simulink model "Simple_CameraInputDisplay_UCS"  (R2025b)
settings: Solver=FixedStepDiscrete  StartTime=0.0  StopTime=inf  FixedStep=.01  RelTol=1e-3
model workspace (MAT data in the model file):
  socvcb = containers.Map
  socvcb.serialization.keys = {}
  socvcb.serialization.values = {}
  socvcb.serialization.uniformity = 0
  socvcb.serialization.keyType = 'double'
  socvcb.serialization.valueType = 'any'
undefined symbols (not defined in the file): distort_coefL, gate1_Pose, gray, k_L, keyPointsWorld, M_UCSToWorld, M_WorldToUCS, numKeypoints, rel_CamPose_L, rel_CamPose_L_UCS, rel_CamPose_R_UCS, Sim3dSensor
libraries: sim3dlib x3, sim3dcameralib x2, visionsinks x2, visiontextngfix x1, visionconversions x1
settings Model: Creator=Liam  LastModifiedBy=Liam

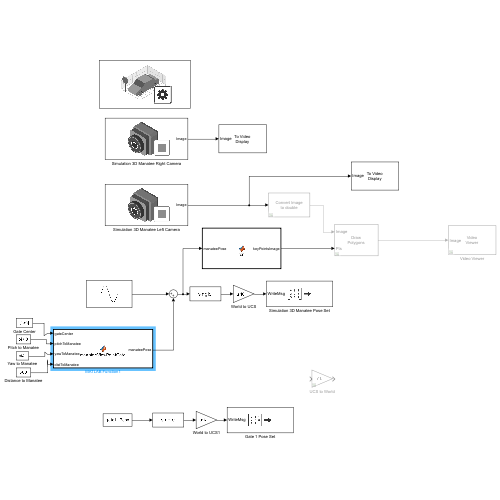
[thumbnail: Simulink's stored preview of the top-level diagram]
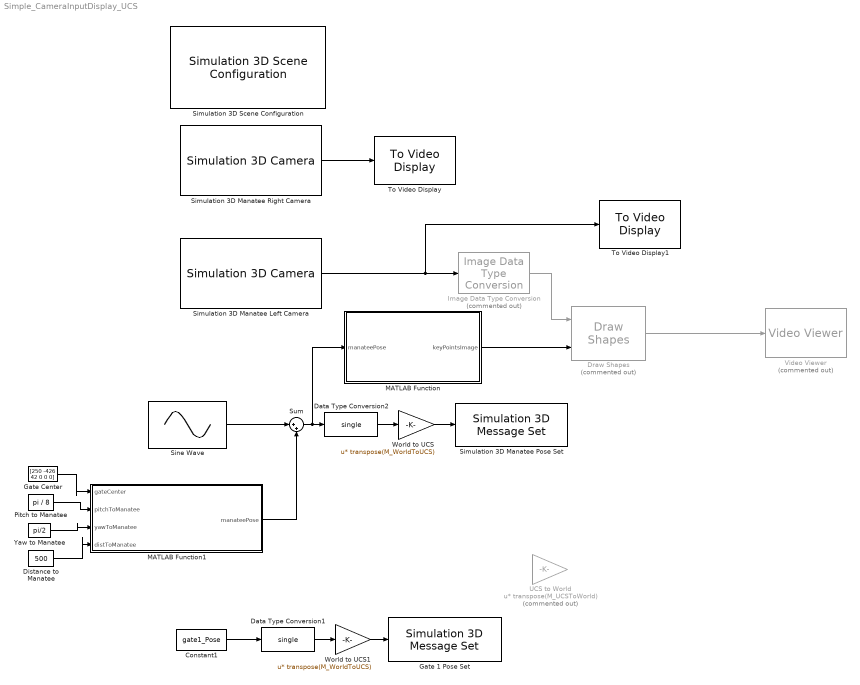
== system Simple_CameraInputDisplay_UCS ==
  Constant1 : Constant  Value=gate1_Pose  VectorParams1D=off  OutDataTypeStr=single
  Data Type Conversion1 : DataTypeConversion  OutDataTypeStr=single  SaturateOnIntegerOverflow=off  RndMeth=Floor
  Data Type Conversion2 : DataTypeConversion  OutDataTypeStr=single  SaturateOnIntegerOverflow=off  RndMeth=Floor
  Distance to Manatee : Constant  Value=500
  Draw Shapes : visiontextngfix/Draw Shapes  Commented=on  shape=Polygons  fill=off  lineWidth=2  fillClrSource=Specify via dialog  display=User-specified value  intensity=200  color=[255 255 0]  opacity=0.6  viewport=Entire image  antialiasing=off  inType=Obsolete  imagePorts=One multidimensional signal  roundingMode=Floor  overflowMode=off  memoryMode=Specify word length  memoryWordLength=16  prodOutputMode=Binary point scaling  prodOutputWordLength=32  prodOutputFracLength=14  memoryFracLength=15
  Gate 1 Pose Set : sim3dlib/Simulation 3D Message Set  Priority=-1  SigName=Gate1PoseSet  Ts=-1  aMode=0
      settings: LibrarySourceBlock=aerolibsim3d/Simulation 3D Message Set
  Gate Center : Constant  Value=[250 -426 42 0 0 0]  VectorParams1D=off  OutDataTypeStr=single
  Image Data Type Conversion : visionconversions/Image Data Type Conversion  Commented=on  outDT=double  isSigned=on  wordLen=16  numFracBits=0
  MATLAB Function : MATLAB Function  TreatAsAtomicUnit=on
  MATLAB Function1 : MATLAB Function  TreatAsAtomicUnit=on
  Pitch to Manatee : Constant  Value=pi / 8
  Simulation 3D Manatee Left Camera : sim3dcameralib/Simulation 3D Camera  Priority=1  sensorTag=Sim3dSensor�  sensorId=1  sensorName=Sim3dSensor�  vehTagList={'Scene Origin'}  vehTag=Scene Origin  CoordinateSystem=Default  mountLoc=Origin  offsetFlag=on  tmountOffset=rel_CamPose_L_UCS(1:3) / 100  extTmount=off  rmountOffset=rel_CamPose_L_UCS(4:6)  extRmount=off  FocalLength=[2.97 / 0.0028, 2.97 / 0.0028]  OpticalCenter=[960, 540]  ImageSize=[1080, 1920]  RadialDistortion=[0.30 0.08]  TangentialDistortion=[0 0]  SensorSkew=0  VisualizeFieldOfView=off  FieldOfViewRange=61  DepthOutportEnabled=off  SemanticOutportEnabled=off  TransformOutportEnabled=off  SampleTime=-1  mountPoint=[0.4 -0.125 -0.15]  mountOrientation=[0 0 0]  aMode=5  ID=1
      settings: LibrarySourceBlock=sl3dlib/Simulation 3D/Sensors/Simulation 3D Camera
  Simulation 3D Manatee Pose Set : sim3dlib/Simulation 3D Message Set  Priority=-1  SigName=ManateePoseSet  Ts=-1  aMode=0
      settings: LibrarySourceBlock=aerolibsim3d/Simulation 3D Message Set
  Simulation 3D Manatee Right Camera : sim3dcameralib/Simulation 3D Camera  Priority=1  sensorTag=Sim3dSensor�  sensorId=2  sensorName=Sim3dSensor�  vehTagList={'Scene Origin'}  vehTag=Scene Origin  CoordinateSystem=Default  mountLoc=Origin  offsetFlag=on  tmountOffset=rel_CamPose_R_UCS(1:3) / 100  extTmount=off  rmountOffset=rel_CamPose_R_UCS(4:6)  extRmount=off  FocalLength=[2.97 / 0.0028, 2.97 / 0.0028]  OpticalCenter=[960, 540]  ImageSize=[1080, 1920]  RadialDistortion=[0.30 0.08]  TangentialDistortion=[0 0]  SensorSkew=0  VisualizeFieldOfView=off  FieldOfViewRange=61  DepthOutportEnabled=off  SemanticOutportEnabled=off  TransformOutportEnabled=off  SampleTime=-1  mountPoint=[0.4 0.125 -0.15]  mountOrientation=[0 0 0]  aMode=5  ID=2
      settings: LibrarySourceBlock=sl3dlib/Simulation 3D/Sensors/Simulation 3D Camera
  Simulation 3D Scene Configuration : sim3dlib/Simulation 3D Scene Configuration  Priority=0  ProjectFormat=Unreal Executable  SceneDesc=Straight road  ProjectName=C:\Users\Liam\OneDrive\Documents\GitHub\Vision_Sim\Unreal\UnrealProjects\SimulinkCoSimulation\EllingtonPoolSim\Windows\EllingtonPoolSim.exe  ScenePath=/Game/PoolMapQuickWater  UEProjPath=C:\Users\Liam\OneDrive\Documents\GitHub\Vision_Sim\Unreal\UnrealProjects\SimulinkCoSimulation\EllingtonPoolSim\EllingtonPoolSim.uproject  EnableOpenDRIVE=off  vehTagList={'Custom';'Scene Origin'}  vehTag=Scene Origin  AttachedCameraRelativeTranslation=[0 0 0]  FreeCameraDefaultInitialTranslation=[-6, 0, 2]  AttachedCameraRelativeRotation=[0 0 0]  FreeCameraDefaultInitialRotation=[0, -15, 0]  ViewpointName=Custom  FreeCameraInitialTranslation=[0, 0, 0]  ViewpointTranslation=[0 0 0]  FreeCameraInitialRotation=[0, 0, 0]  ViewpointRotation=[0 0 0]  OpVisEn=off  Ts=0.03  EnableWindow=on  EnableRemoteAccess=off  EnableWeather=off  SunAzimuth=90  SunAltitude=40.0  EnableGeospatialSun=off  Latitude=0  Longitude=0  Date=2023-01-01  Time=10:30:00  GeoTimeZone=-5.0  SunDaylightSaving=off  wind=1  clouds=10  EnableVolumetricClouds=off  CloudCoverage=0  CloudAltitude=6  fog=0  rain=0  RaindropsEffect=off  SnowDensity=0  EnableGeospatial=off  TilesetSource=Earth terrain  UseTrueOrigin=off  OriginHeight=200  OriginLatitude=40.744652  OriginLongitude=-73.988864  MapStyle=Aerial  AdditionalAssetIDs=[]  UseAdvancedSunSky=off  SolarTime=11  TimeZone=-5  Day=21  Month=9  Year=2022  UseDaylightSavingTime=on  DSTStartDay=10  DSTStartMonth=3  DSTEndDay=3  DSTEndMonth=11  DSTSwitchHour=2  sensorTag=MainCamera1  sensorId=1  sensorName=MainCamera1  mountLoc=Origin  offsetFlag=off  tmountOffset=[0, 0, 0]  rmountOffset=[0, 0, 0]  HorizontalResolution=1280  VerticalResolution=720  HorizontalFOV=60  mountPoint=[0 0 0]  mountOrientation=[0 0 0]  aMode=3  ID=1  GeoTrigger=Inactive  ViewNameList={'Custom'}  ViewTranslationList={'[0 0 0]'}  ViewRotationList={'[0 0 0]'}
      settings: LibrarySourceBlock=drivingsim3d/Simulation 3D Scene Configuration
  Sine Wave : Sin  Amplitude=[30 30 30 pi/12 0 pi/12]  Frequency=[0.2 0.2 0.4 0.03 0.01 0.05]  Phase=[0 90 0 0 0 0]  SampleTime=0
  Sum : Sum  Inputs=|++
  To Video Display : visionsinks/To Video Display  windowSizeMode=Normal  openAtMdlStart=on  fullScreen=off  videoWindowX=536805376  videoWindowY=536805376  saveWindowSize=off  videoWindowWidth=1920  videoWindowHeight=1080  inputColorFormat=RGB  inputType=Obsolete  imagePorts=One multidimensional signal  OutputDevice=On-screen video monitor  dataOrg=Column-major  isWindowOpen=off
  To Video Display1 : visionsinks/To Video Display  windowSizeMode=Normal  openAtMdlStart=on  fullScreen=off  videoWindowX=536805376  videoWindowY=536805376  saveWindowSize=off  videoWindowWidth=1920  videoWindowHeight=1080  inputColorFormat=RGB  inputType=Obsolete  imagePorts=One multidimensional signal  OutputDevice=On-screen video monitor  dataOrg=Column-major  isWindowOpen=off
  UCS to World : Gain  Commented=on  Gain=transpose(M_UCSToWorld)  Multiplication=Matrix(u*K)
  Video Viewer : VideoViewer  Commented=on  colormapValue=gray(256)  FigPos=[1 910 1536 813]
  World to UCS : Gain  Gain=transpose(M_WorldToUCS)  Multiplication=Matrix(u*K)
  World to UCS1 : Gain  Gain=transpose(M_WorldToUCS)  Multiplication=Matrix(u*K)
  Yaw to Manatee : Constant  Value=pi/2
  wires:
  Data Type Conversion2/1 -> World to UCS/1
  Sine Wave/1 -> Sum/1
  Sum/1 -> MATLAB Function/1(manateePose), Data Type Conversion2/1
  Constant1/1 -> Data Type Conversion1/1
  Data Type Conversion1/1 -> World to UCS1/1
  World to UCS/1 -> Simulation 3D Manatee Pose Set/1
  World to UCS1/1 -> Gate 1 Pose Set/1
  Simulation 3D Manatee Right Camera/1 -> To Video Display/1
  MATLAB Function/1(keyPointsImage) -> Draw Shapes/2
  Image Data Type Conversion/1 -> Draw Shapes/1
  Draw Shapes/1 -> Video Viewer/1
  Simulation 3D Manatee Left Camera/1 -> To Video Display1/1, Image Data Type Conversion/1
  Distance to Manatee/1 -> MATLAB Function1/4(distToManatee)
  Pitch to Manatee/1 -> MATLAB Function1/2(pitchToManatee)
  Yaw to Manatee/1 -> MATLAB Function1/3(yawToManatee)
  Gate Center/1 -> MATLAB Function1/1(gateCenter)
  MATLAB Function1/1(manateePose) -> Sum/2

== matlab function Simple_CameraInputDisplay_UCS/MATLAB Function1 ==
  data: gateCenter input; manateePose output; pitchToManatee input; yawToManatee input; distToManatee input
function manateePose = manateeViewPointGate(gateCenter, pitchToManatee, yawToManatee, distToManatee)
R_M = getRotationMatrix([0 pitchToManatee yawToManatee]);
vector = R_M * [distToManatee; 0; 0; 1];
manateePose = [(gateCenter(1) + vector(1)) (gateCenter(2) + vector(2)) (gateCenter(3) + vector(3)) 0 -pitchToManatee  (yawToManatee + pi)];

== matlab function Simple_CameraInputDisplay_UCS/MATLAB Function ==
  data: manateePose input; rel_CamPose_L parameter; keyPointsWorld parameter; k_L parameter; distort_coefL parameter; numKeypoints parameter; keyPointsImage output
function keyPointsImage = fcn(manateePose,rel_CamPose_L, keyPointsWorld, k_L, distort_coefL, numKeypoints)
keyPointsImageList = zeros(numKeypoints,2);
keyPointsImage = zeros(1,8);
for i = 1:numKeypoints
    keyPoint = worldToImageCoord(keyPointsWorld(i,:), manateePose, rel_CamPose_L, k_L, distort_coefL);
    keyPointsImageList(i,:) = keyPoint(:);
    keyPointsImage(2*i - 1) = keyPoint(1);
    keyPointsImage(2*i) = keyPoint(2);
end
